simulink library "BLOM_Lib"  (Simulink 7.4)
settings: Solver=ode45  StartTime=0.0  StopTime=10.0  MaxStep=0.01  RelTol=1e-3
values from neighbouring files (symbols this model uses):
  simin = [0 1]    [testscript.m]
undefined symbols (not defined in the file or in its folder): sparse
libraries: BLOM_Lib x2
settings Model: Creator=JJK  LastModifiedBy=Kyle

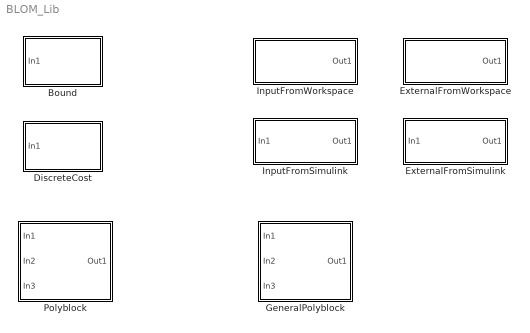
== system BLOM_Lib ==
  Bound : Subsystem  mask{ub=inf, lb=-inf, initial_step=on, final_step=on, intermediate_step=on}
      mask prompts: ub "Upper bound:"; lb "Lower bound:"; initial_step "Apply at the initial time step?"; final_step "Apply at the final time step?"; intermediate_step "Apply at all other time steps?"
      mask help: Please specify the upper and lower bounds of this variable.
      mask Display: fprintf('Bound')
  DiscreteCost : Subsystem  mask{initial_step=on, final_step=on, intermediate_step=on}
      mask prompts: initial_step "Does signal add to cost at the initial time step?"; final_step "Does signal add to cost at the final time step?"; intermediate_step "Does signal add to cost at all other time steps?"
      mask Display: fprintf('Discrete Cost')
  ExternalFromSimulink : Subsystem  mask{interpType=Zero-Order Hold}
      mask prompts: interpType "Interpolation type"
      mask StyleString: popup(Zero-Order Hold|First-Order Hold)
      mask Display: fprintf('External')
  ExternalFromWorkspace : Subsystem  mask{simin=simin, interpType=Zero-Order Hold}
      mask prompts: simin "Data:"; interpType "Interpolation type"
      mask help:
      | Read data values specified in matrix or structure format from MATLAB's workspace.
      |
      | Matrix format can be used only for one-dimensional signals. Each row of the matrix has a time stamp in the first column and a vector containing the corresponding data sample in the subsequent column(s).
      |
      | Structure format can be used for either one-dimensional or multidimensional signals:
      |     var.time=[TimeValues]
      |     var.signals.values=[DataValues]
      |     var.signals.dimensions=[DimValues]
      mask StyleString: edit,popup(Zero-Order Hold|First-Order Hold)
      mask Display: fprintf('External')
  GeneralPolyblock : Subsystem  mask{P_f=sparse([1 1 0; 3 1 0]), K_f=sparse([1 0.8]), P_g=[0 0 0], K_g=[1], inputs=x1,x2,x3, inputScalar=on, outputScalar=on}
      mask prompts: P_f "P matrix f(X)"; K_f "K matrix f(x)"; P_g "P matrix g(x)"; K_g "K matrix g(x)"; inputs "Input names, comma separated"; inputScalar "Input(s) as scalar?"; outputScalar "Output(s) as scalar?"
      mask help:
      | y = f(x)/g(x)
      | where f and g are a sum of polynomial and exponential terms, described by P and K matricies.
      | Example: f=x1*exp(x3)+0.8x1^3*x2
      | P_f = [1 0 BLOM_FunctionCode('exp');
      |      3 1 0];
      | K_f = [1 0.8];
      mask init:
      | BLOM_PolyblockChangeInputs(gcb,P_f,K_f,inputs,inputScalar,outputScalar)
      | 
      | if (size(P_f,2) ~= size(P_g,2))
      |     str =[gcb ': Number of columns of P in f must be equal to number of columns of P in g!']; 
      |     disp(str);
      |     error(str);
      | end
      | 
      | if (size(P_f,1) ~= size(K_f,2))
      |     str =[gcb ': Number of rows of P in f must be equal to number of columns of K in f!'];
      |     disp(str);
      |     error(str);
      | end
      | 
      | if (size(P_g,1) ~= size(K_g,2))
      |     str =[gcb ': Number of rows of P in g must be equal to number of columns of K in g!'];
      |     disp(str);
      |     error(str);
      | end
      | 
      | if (size(K_g,1) ~= 1 && size(K_g,1) ~= size(K_f,1))
      |     str =[gcb ': g must be a scalar function or equal dimension to f'];
      |     disp(str);
      |     error(str);
      | end
      mask Display: fprintf('Polyblock f(x)/g(x)')
  InputFromSimulink : Subsystem  mask{interpType=Zero-Order Hold}
      mask prompts: interpType "Interpolation type"
      mask StyleString: popup(Zero-Order Hold|First-Order Hold)
      mask Display: fprintf('Input')
  InputFromWorkspace : Subsystem  mask{simin=simin, interpType=Zero-Order Hold}
      mask prompts: simin "Data:"; interpType "Interpolation type"
      mask help:
      | Read data values specified in matrix or structure format from MATLAB's workspace.
      |
      | Matrix format can be used only for one-dimensional signals. Each row of the matrix has a time stamp in the first column and a vector containing the corresponding data sample in the subsequent column(s).
      |
      | Structure format can be used for either one-dimensional or multidimensional signals:
      |     var.time=[TimeValues]
      |     var.signals.values=[DataValues]
      |     var.signals.dimensions=[DimValues]
      mask StyleString: edit,popup(Zero-Order Hold|First-Order Hold)
      mask Display: fprintf('Input')
  Polyblock : Subsystem  mask{P=sparse([1 1 0; 3 1 0]), K=sparse([1 0.8]), inputs=x1,x2, inputScalar=on, outputScalar=on}
      mask prompts: P "P matrix"; K "K matrix"; inputs "Input names, comma separated"; inputScalar "Input(s) as scalar?"; outputScalar "Output(s) as scalar?"
      mask help:
      | y = f(x)
      | where f is a sum of polynomial and exponential terms, described by P and K matricies.
      | Example: f=x1*exp(x3)+0.8x1^3*x2
      | P = [1 0 BLOM_FunctionCode('exp');
      |      3 1 0];
      | K = [1 0.8];
      mask init:
      | BLOM_PolyblockChangeInputs(gcb,P,K,inputs,inputScalar,outputScalar)
      mask Display: fprintf('Polyblock')

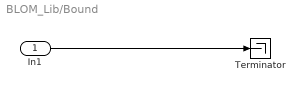
== system BLOM_Lib/Bound ==
  In1 : Inport
  Terminator : Terminator
  wires:
  In1/1 -> Terminator/1

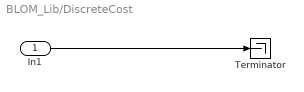
== system BLOM_Lib/DiscreteCost ==
  In1 : Inport
  Terminator : Terminator
  wires:
  In1/1 -> Terminator/1

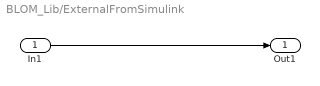
== system BLOM_Lib/ExternalFromSimulink ==
  In1 : Inport  OutDataType=fixdt(1, 16)  OutScaling=2^0
  Out1 : Outport  OutDataType=fixdt(1, 16)  OutScaling=2^0
  wires:
  In1/1 -> Out1/1

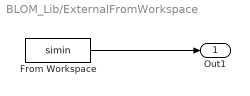
== system BLOM_Lib/ExternalFromWorkspace ==
  From Workspace : FromWorkspace  VariableName=simin  SampleTime=0
  Out1 : Outport  OutDataType=fixdt(1, 16)  OutScaling=2^0
  wires:
  From Workspace/1 -> Out1/1

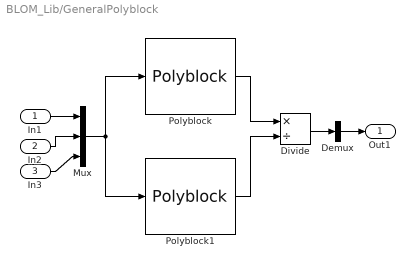
== system BLOM_Lib/GeneralPolyblock ==
  In1 : Inport  OutDataType=fixdt(1, 16)  OutScaling=2^0
  In2 : Inport  Port=2  OutDataType=fixdt(1, 16)  OutScaling=2^0
  In3 : Inport  Port=3  OutDataType=fixdt(1, 16)  OutScaling=2^0
  Demux : Demux  Outputs=1
  Divide : Product  Inputs=*/  OutDataType=fixdt(1, 16)  OutScaling=2^-10
  Mux : Mux  Inputs=3
  Polyblock : BLOM_Lib/Polyblock  SystemSampleTime=-1  P=P_f  K=K_f  inputs=x  inputScalar=off  outputScalar=off
  Polyblock1 : BLOM_Lib/Polyblock  SystemSampleTime=-1  P=P_g  K=K_g  inputs=x  inputScalar=off  outputScalar=off
  Out1 : Outport  OutDataType=fixdt(1, 16)  OutScaling=2^0
  wires:
  In1/1 -> Mux/1
  Demux/1 -> Out1/1
  In2/1 -> Mux/2
  In3/1 -> Mux/3
  Mux/1 -> Polyblock/1, Polyblock1/1
  Polyblock/1 -> Divide/1
  Polyblock1/1 -> Divide/2
  Divide/1 -> Demux/1

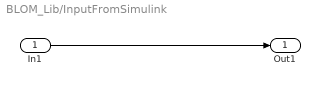
== system BLOM_Lib/InputFromSimulink ==
  In1 : Inport  OutDataType=fixdt(1, 16)  OutScaling=2^0
  Out1 : Outport  OutDataType=fixdt(1, 16)  OutScaling=2^0
  wires:
  In1/1 -> Out1/1

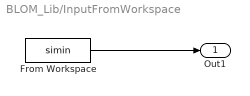
== system BLOM_Lib/InputFromWorkspace ==
  From Workspace : FromWorkspace  VariableName=simin  SampleTime=0
  Out1 : Outport  OutDataType=fixdt(1, 16)  OutScaling=2^0
  wires:
  From Workspace/1 -> Out1/1

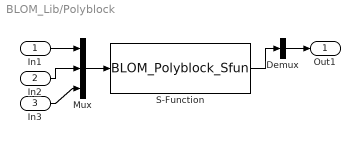
== system BLOM_Lib/Polyblock ==
  In1 : Inport  OutDataType=fixdt(1, 16)  OutScaling=2^0
  In2 : Inport  Port=2  OutDataType=fixdt(1, 16)  OutScaling=2^0
  In3 : Inport  Port=3  OutDataType=fixdt(1, 16)  OutScaling=2^0
  Demux : Demux  Outputs=1
  Mux : Mux  Inputs=3
  S-Function : S-Function  FunctionName=BLOM_Polyblock_Sfun  Parameters=P,K  EnableBusSupport=off
  Out1 : Outport  OutDataType=fixdt(1, 16)  OutScaling=2^0
  wires:
  In1/1 -> Mux/1
  Demux/1 -> Out1/1
  In2/1 -> Mux/2
  Mux/1 -> S-Function/1
  S-Function/1 -> Demux/1
  In3/1 -> Mux/3
